simulink model "LDW_mask"  (Simulink 7.6)
settings: Solver=FixedStepDiscrete  StartTime=0.0  StopTime=10  FixedStep=1/100  RelTol=1e-3
undefined symbols (not defined in the file): High, num_targets, slselsubs
libraries: simulink x36, dspobslib x14, viptextngfix x9, dspmtrx3 x7, dspsigops x6, simulink_extras x4, viptransforms x4, dspstat3 x4, dspswit3 x3, dspadpt3 x3, dspindex x2, vipconversions x2
(part 3 of 3)

== system LDW_mask/LDW Model/Subsystem1/Lane Detection/Peak detection/Enable signal generator ==
  Num : Inport
  Assignment : Assignment  NumberOfDimensions=2  IndexOptions=Assign all,Index vector (port)  Indices=-1,1  OutputSizes=1,1
  Constant : Constant  Value=zeros(1, expLaneNum)  VectorParams1D=off  OutDataTypeStr=boolean
  Constant1 : Constant  VectorParams1D=off  OutDataTypeStr=boolean
  For Iterator : ForIterator  ResetStates=reset  IterationSource=external
  Enable : Outport
  wires:
  For Iterator/1 -> Assignment/3
  Constant1/1 -> Assignment/2
  Assignment/1 -> Enable/1
  Constant/1 -> Assignment/1
  Num/1 -> For Iterator/1

== system LDW_mask/LDW Model/Subsystem1/Lane Detection/Peak detection1/Enable signal generator ==
  Num : Inport
  Assignment : Assignment  NumberOfDimensions=2  IndexOptions=Assign all,Index vector (port)  Indices=-1,1  OutputSizes=1,1
  Constant : Constant  Value=zeros(1, expLaneNum)  VectorParams1D=off  OutDataTypeStr=boolean
  Constant1 : Constant  VectorParams1D=off  OutDataTypeStr=boolean
  For Iterator : ForIterator  ResetStates=reset  IterationSource=external
  Enable : Outport
  wires:
  Num/1 -> For Iterator/1
  Constant/1 -> Assignment/1
  Assignment/1 -> Enable/1
  Constant1/1 -> Assignment/2
  For Iterator/1 -> Assignment/3

== system LDW_mask/LDW Model/Subsystem1/Lane Tracking/Matching/Calculate the distances between  the lines found in the current  frame and those in the respository ==
  Count : Inport
  Rep_ref : Inport  Port=2
  Line : Inport  Port=3
  Enable : Inport  Port=4
  For Iterator : ForIterator  ResetStates=reset  IterationLimit=maxLaneNum
  "Select a line from the repository; if it is valid (Count > 0),  Calculate its distance to the input lines." : Subsystem
  Selector1 : Selector  NumberOfDimensions=2  InputPortWidth=3  IndexOptions=Select all,Index vector (port)  Indices=-1,-1  OutputSizes=1
  Dis : Outport
  wires:
  Enable/1 -> "Select a line from the repository; if it is valid (Count > 0),  Calculate its distance to the input lines."/4(Enable)
  For Iterator/1 -> Selector1/2, "Select a line from the repository; if it is valid (Count > 0),  Calculate its distance to the input lines."/1(Idx)
  "Select a line from the repository; if it is valid (Count > 0),  Calculate its distance to the input lines."/1(Dis) -> Dis/1
  Rep_ref/1 -> "Select a line from the repository; if it is valid (Count > 0),  Calculate its distance to the input lines."/2(Rep_ref)
  Line/1 -> "Select a line from the repository; if it is valid (Count > 0),  Calculate its distance to the input lines."/3(Line)
  Count/1 -> Selector1/1
  Selector1/1 -> "Select a line from the repository; if it is valid (Count > 0),  Calculate its distance to the input lines."/Enable

== system LDW_mask/LDW Model/Subsystem1/Lane Tracking/Matching/Find the best  matches between the current  lines and those in the repository ==
  note: In the 1st iteration, find minimum element (corresponds to
      | best matching targets) in the distance matrix. Then, use the
      | updated distance matrix where the minimum elements and
      | their  corresponding rows and columns have been reset.
  note: Reset the column where the
      | minimum element lies on.
  note: Reset the row where the
      | minimum element lies on.
  Dis : Inport
  Add : Sum
  Assignment : Assignment  NumberOfDimensions=2  IndexOptions=Assign all,Index vector (port)  Indices=-1,-1  OutputSizes=1,1
  Assignment1 : Assignment  NumberOfDimensions=2  IndexOptions=Index vector (port),Assign all  Indices=1,-1  OutputSizes=1,1
  Assignment2 : Assignment  NumberOfDimensions=2  IndexOptions=Assign all,Index vector (port)  Indices=-1,-1  OutputSizes=1,1
  Assignment3 : Assignment  NumberOfDimensions=2  IndexOptions=Assign all,Index vector (port)  Indices=-1,-1  OutputSizes=1,1
  Compare To Constant : simulink/Logic and Bit Operations/Compare To Constant  SystemSampleTime=-1  relop=<=  const=1  LogicOutDataTypeMode=boolean  ZeroCross=off
  Constant : Constant  Value=intmax('int16')  VectorParams1D=off  OutDataTypeStr=Inherit: Inherit via back propagation
  Constant1 : Constant  Value=intmax('int16')*ones(1,maxLaneNum, 'int16')  VectorParams1D=off  OutDataTypeStr=Inherit: Inherit via back propagation
  Constant2 : Constant  Value=zeros(2,maxLaneNum)  VectorParams1D=off  OutDataTypeStr=Inherit: Inherit via back propagation
  Data Type  Conversion3 : DataTypeConversion  OutDataTypeStr=int32  SaturateOnIntegerOverflow=on  RndMeth=Zero
  Delay1 : dspsigops/Delay  dly_unit=Samples  delay=1  ic_detail=off  dif_ic_for_ch=off  dif_ic_for_dly=off  ic=0  reset_popup=None
  For Iterator : ForIterator  IterationLimit=expLaneNum
  Minimum : dspstat3/Minimum  DialogController=dspDDGCreate  DialogControllerArgs=DataTag11  fcn=Value and Index  reset=None  indexBase=One  operateOver=Entire input  Dimension=1  colComp=on  operation=minimum  roiEnable=off  roiType=Rectangles  roiPortion=Entire ROI  roiOutput=Individual statistics for each ROI  roiFlag=off  roundingMode=Floor  overflowMode=off
  Reshape : Reshape  OutputDimensionality=Column vector (2-D)
  Selector : Selector  InputPortWidth=2  IndexOptions=Index vector (dialog)  Indices=[2]  OutputSizes=1
  Selector1 : Selector  InputPortWidth=2  IndexOptions=Index vector (dialog)  Indices=[1]  OutputSizes=1
  Switch1 : Switch  Criteria=u2 ~= 0
  Match_list : Outport
  Match_dis : Outport  Port=2
  wires:
  Constant2/1 -> Assignment/1
  Constant1/1 -> Assignment3/1
  Data Type  Conversion3/1 -> Reshape/1
  Compare To Constant/1 -> Switch1/2
  For Iterator/1 -> Compare To Constant/1, Assignment/3, Assignment3/3
  Switch1/1 -> Minimum/1
  Dis/1 -> Assignment2/1, Assignment1/1, Switch1/1
  Delay1/1 -> Switch1/3
  Assignment/1 -> Match_list/1
  Selector/1 -> Assignment2/3
  Selector1/1 -> Assignment1/3
  Assignment1/1 -> Add/1
  Assignment2/1 -> Add/2
  Add/1 -> Delay1/1
  Assignment3/1 -> Match_dis/1
  Minimum/2 -> Data Type  Conversion3/1, Selector/1, Selector1/1
  Minimum/1 -> Assignment3/2
  Constant/1 -> Assignment1/2, Assignment2/2
  Reshape/1 -> Assignment/2

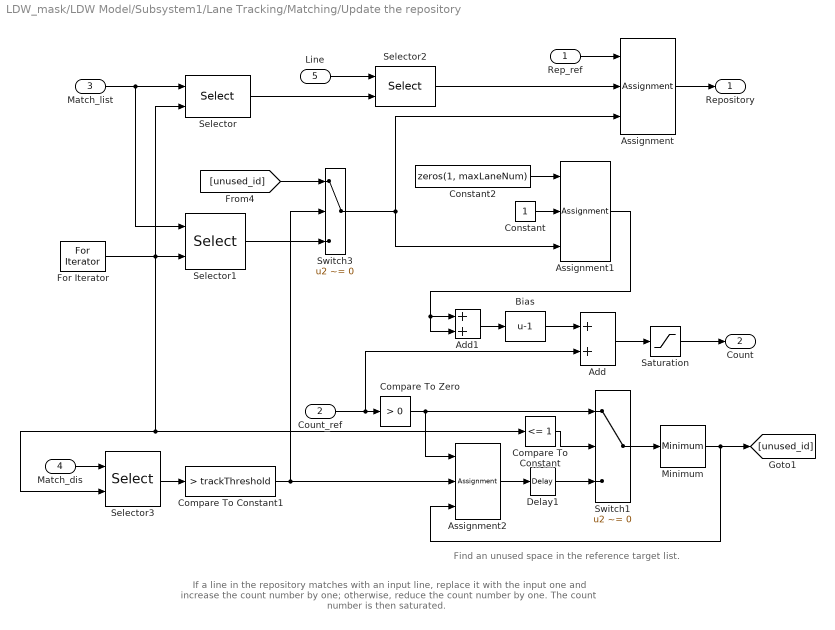
== system LDW_mask/LDW Model/Subsystem1/Lane Tracking/Matching/Update the repository ==
  note: Find an unused space in the reference target list.
  note: If a line in the repository matches with an input line, replace it with the input one and increase the count number by one;
      | otherwise, reduce the count number by one. The count number is then saturated.
  Rep_ref : Inport
  Count_ref : Inport  Port=2
  Match_list : Inport  Port=3
  Match_dis : Inport  Port=4
  Line : Inport  Port=5
  Add : Sum  InputSameDT=on
  Add1 : Sum  OutDataTypeStr=int32  InputSameDT=on
  Assignment : Assignment  NumberOfDimensions=2  IndexOptions=Assign all,Starting index (port)  Indices=-1,-1  OutputSizes=1,1
  Assignment1 : Assignment  NumberOfDimensions=2  IndexOptions=Assign all,Index vector (port)  Indices=-1,-1  OutputSizes=slselsubs([1, num_targets],1),slselsubs([1, num_targets],2)
  Assignment2 : Assignment  IndexOptions=Index vector (port)  Indices=-1  OutputSizes=[1, num_targets]
  Bias : Bias  Bias=-1
  Compare To Constant : simulink/Logic and Bit Operations/Compare To Constant  SystemSampleTime=-1  relop=<=  const=1  LogicOutDataTypeMode=boolean  ZeroCross=off
  Compare To Constant1 : simulink/Logic and Bit Operations/Compare To Constant  SystemSampleTime=-1  relop=>  const=trackThreshold  LogicOutDataTypeMode=boolean  ZeroCross=off
  Compare To Zero : simulink/Logic and Bit Operations/Compare To Zero  SystemSampleTime=-1  relop=>  LogicOutDataTypeMode=boolean  ZeroCross=off
  Constant : Constant  VectorParams1D=off  OutDataTypeStr=Inherit: Inherit via back propagation
  Constant2 : Constant  Value=zeros(1, maxLaneNum)  VectorParams1D=off  OutDataTypeStr=int32
  Delay1 : dspsigops/Delay  dly_unit=Samples  delay=1  ic_detail=off  dif_ic_for_ch=off  dif_ic_for_dly=off  ic=0  reset_popup=None
  For Iterator : ForIterator  ResetStates=reset  IterationLimit=expLaneNum
  Minimum : dspstat3/Minimum  DialogController=dspDDGCreate  DialogControllerArgs=DataTag12  fcn=Index  reset=None  indexBase=One  operateOver=Each row  Dimension=1  colComp=on  operation=minimum  roiEnable=off  roiType=Rectangles  roiPortion=Entire ROI  roiOutput=Individual statistics for each ROI  roiFlag=off  roundingMode=Floor  overflowMode=off
  Saturation : Saturate  UpperLimit=frameFound+frameLost  LowerLimit=0
  Selector : Selector  NumberOfDimensions=2  InputPortWidth=3  IndexOptions=Index vector (dialog),Index vector (port)  Indices=[2],[1]  OutputSizes=1
  Selector1 : Selector  NumberOfDimensions=2  InputPortWidth=3  IndexOptions=Index vector (dialog),Index vector (port)  Indices=[1],[2]  OutputSizes=1
  Selector2 : Selector  NumberOfDimensions=2  InputPortWidth=3  IndexOptions=Select all,Index vector (port)  Indices=-1,1  OutputSizes=1
  Selector3 : Selector  NumberOfDimensions=2  InputPortWidth=3  IndexOptions=Select all,Index vector (port)  Indices=-1,-1  OutputSizes=1
  Switch1 : Switch  Criteria=u2 ~= 0
  Switch3 : Switch  Criteria=u2 ~= 0
  Repository : Outport
  Count : Outport  Port=2
  wires:
  Constant2/1 -> Assignment1/1
  Constant/1 -> Assignment1/2
  Switch3/1 -> Assignment1/3, Assignment/3
  Selector1/1 -> Switch3/3
  Selector/1 -> Selector2/2
  [unused_id] -> Switch3/1
  Compare To Constant1/1 -> Switch3/2, Assignment2/2
  Delay1/1 -> Switch1/3
  Count_ref/1 -> Add/2, Compare To Zero/1
  Switch1/1 -> Minimum/1
  Minimum/1 -> [unused_id], Assignment2/3
  Assignment2/1 -> Delay1/1
  Match_dis/1 -> Selector3/1
  Assignment1/1 -> Add1/1, Add1/2
  Assignment/1 -> Repository/1
  Line/1 -> Selector2/1
  Match_list/1 -> Selector/1, Selector1/1
  Compare To Constant/1 -> Switch1/2
  For Iterator/1 -> Selector3/2, Compare To Constant/1, Selector/2, Selector1/2
  Selector2/1 -> Assignment/2
  Add1/1 -> Bias/1
  Bias/1 -> Add/1
  Add/1 -> Saturation/1
  Compare To Zero/1 -> Switch1/1, Assignment2/1
  Rep_ref/1 -> Assignment/1
  Selector3/1 -> Compare To Constant1/1
  Saturation/1 -> Count/1

== system LDW_mask/LDW Model/Subsystem1/Lane Tracking1/Matching/Calculate the distances between  the lines found in the current  frame and those in the respository ==
  Count : Inport
  Rep_ref : Inport  Port=2
  Line : Inport  Port=3
  Enable : Inport  Port=4
  For Iterator : ForIterator  ResetStates=reset  IterationLimit=maxLaneNum
  "Select a line from the repository; if it is valid (Count > 0),  Calculate its distance to the input lines." : Subsystem
  Selector1 : Selector  NumberOfDimensions=2  InputPortWidth=3  IndexOptions=Select all,Index vector (port)  Indices=-1,-1  OutputSizes=1
  Dis : Outport
  wires:
  Selector1/1 -> "Select a line from the repository; if it is valid (Count > 0),  Calculate its distance to the input lines."/Enable
  Count/1 -> Selector1/1
  Line/1 -> "Select a line from the repository; if it is valid (Count > 0),  Calculate its distance to the input lines."/3(Line)
  Rep_ref/1 -> "Select a line from the repository; if it is valid (Count > 0),  Calculate its distance to the input lines."/2(Rep_ref)
  "Select a line from the repository; if it is valid (Count > 0),  Calculate its distance to the input lines."/1(Dis) -> Dis/1
  For Iterator/1 -> "Select a line from the repository; if it is valid (Count > 0),  Calculate its distance to the input lines."/1(Idx), Selector1/2
  Enable/1 -> "Select a line from the repository; if it is valid (Count > 0),  Calculate its distance to the input lines."/4(Enable)

== system LDW_mask/LDW Model/Subsystem1/Lane Tracking1/Matching/Find the best  matches between the current  lines and those in the repository ==
  note: Reset the row where the
      | minimum element lies on.
  note: Reset the column where the
      | minimum element lies on.
  note: In the 1st iteration, find minimum element (corresponds to
      | best matching targets) in the distance matrix. Then, use the
      | updated distance matrix where the minimum elements and
      | their  corresponding rows and columns have been reset.
  Dis : Inport
  Add : Sum
  Assignment : Assignment  NumberOfDimensions=2  IndexOptions=Assign all,Index vector (port)  Indices=-1,-1  OutputSizes=1,1
  Assignment1 : Assignment  NumberOfDimensions=2  IndexOptions=Index vector (port),Assign all  Indices=1,-1  OutputSizes=1,1
  Assignment2 : Assignment  NumberOfDimensions=2  IndexOptions=Assign all,Index vector (port)  Indices=-1,-1  OutputSizes=1,1
  Assignment3 : Assignment  NumberOfDimensions=2  IndexOptions=Assign all,Index vector (port)  Indices=-1,-1  OutputSizes=1,1
  Compare To Constant : simulink/Logic and Bit Operations/Compare To Constant  SystemSampleTime=-1  relop=<=  const=1  LogicOutDataTypeMode=boolean  ZeroCross=off
  Constant : Constant  Value=intmax('int16')  VectorParams1D=off  OutDataTypeStr=Inherit: Inherit via back propagation
  Constant1 : Constant  Value=intmax('int16')*ones(1,maxLaneNum, 'int16')  VectorParams1D=off  OutDataTypeStr=Inherit: Inherit via back propagation
  Constant2 : Constant  Value=zeros(2,maxLaneNum)  VectorParams1D=off  OutDataTypeStr=Inherit: Inherit via back propagation
  Data Type  Conversion3 : DataTypeConversion  OutDataTypeStr=int32  SaturateOnIntegerOverflow=on  RndMeth=Zero
  Delay1 : dspsigops/Delay  dly_unit=Samples  delay=1  ic_detail=off  dif_ic_for_ch=off  dif_ic_for_dly=off  ic=0  reset_popup=None
  For Iterator : ForIterator  IterationLimit=expLaneNum
  Minimum : dspstat3/Minimum  DialogController=dspDDGCreate  DialogControllerArgs=DataTag14  fcn=Value and Index  reset=None  indexBase=One  operateOver=Entire input  Dimension=1  colComp=on  operation=minimum  roiEnable=off  roiType=Rectangles  roiPortion=Entire ROI  roiOutput=Individual statistics for each ROI  roiFlag=off  roundingMode=Floor  overflowMode=off
  Reshape : Reshape  OutputDimensionality=Column vector (2-D)
  Selector : Selector  InputPortWidth=2  IndexOptions=Index vector (dialog)  Indices=[2]  OutputSizes=1
  Selector1 : Selector  InputPortWidth=2  IndexOptions=Index vector (dialog)  Indices=[1]  OutputSizes=1
  Switch1 : Switch  Criteria=u2 ~= 0
  Match_list : Outport
  Match_dis : Outport  Port=2
  wires:
  Reshape/1 -> Assignment/2
  Constant/1 -> Assignment2/2, Assignment1/2
  Minimum/1 -> Assignment3/2
  Minimum/2 -> Selector1/1, Selector/1, Data Type  Conversion3/1
  Assignment3/1 -> Match_dis/1
  Add/1 -> Delay1/1
  Assignment2/1 -> Add/2
  Assignment1/1 -> Add/1
  Selector1/1 -> Assignment1/3
  Selector/1 -> Assignment2/3
  Assignment/1 -> Match_list/1
  Delay1/1 -> Switch1/3
  Dis/1 -> Switch1/1, Assignment1/1, Assignment2/1
  Switch1/1 -> Minimum/1
  For Iterator/1 -> Assignment3/3, Assignment/3, Compare To Constant/1
  Compare To Constant/1 -> Switch1/2
  Data Type  Conversion3/1 -> Reshape/1
  Constant1/1 -> Assignment3/1
  Constant2/1 -> Assignment/1

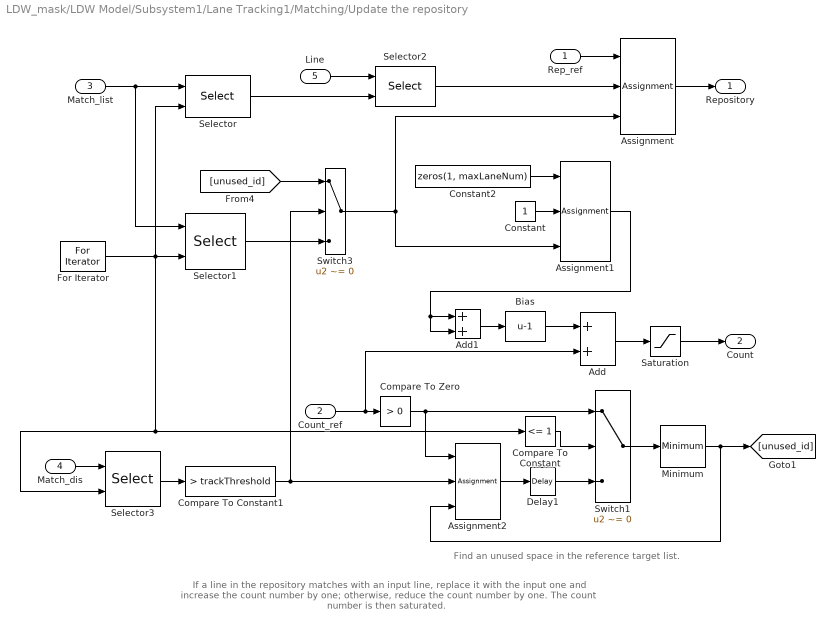
== system LDW_mask/LDW Model/Subsystem1/Lane Tracking1/Matching/Update the repository ==
  note: If a line in the repository matches with an input line, replace it with the input one and increase the count number by one;
      | otherwise, reduce the count number by one. The count number is then saturated.
  note: Find an unused space in the reference target list.
  Rep_ref : Inport
  Count_ref : Inport  Port=2
  Match_list : Inport  Port=3
  Match_dis : Inport  Port=4
  Line : Inport  Port=5
  Add : Sum  InputSameDT=on
  Add1 : Sum  OutDataTypeStr=int32  InputSameDT=on
  Assignment : Assignment  NumberOfDimensions=2  IndexOptions=Assign all,Starting index (port)  Indices=-1,-1  OutputSizes=1,1
  Assignment1 : Assignment  NumberOfDimensions=2  IndexOptions=Assign all,Index vector (port)  Indices=-1,-1  OutputSizes=slselsubs([1, num_targets],1),slselsubs([1, num_targets],2)
  Assignment2 : Assignment  IndexOptions=Index vector (port)  Indices=-1  OutputSizes=[1, num_targets]
  Bias : Bias  Bias=-1
  Compare To Constant : simulink/Logic and Bit Operations/Compare To Constant  SystemSampleTime=-1  relop=<=  const=1  LogicOutDataTypeMode=boolean  ZeroCross=off
  Compare To Constant1 : simulink/Logic and Bit Operations/Compare To Constant  SystemSampleTime=-1  relop=>  const=trackThreshold  LogicOutDataTypeMode=boolean  ZeroCross=off
  Compare To Zero : simulink/Logic and Bit Operations/Compare To Zero  SystemSampleTime=-1  relop=>  LogicOutDataTypeMode=boolean  ZeroCross=off
  Constant : Constant  VectorParams1D=off  OutDataTypeStr=Inherit: Inherit via back propagation
  Constant2 : Constant  Value=zeros(1, maxLaneNum)  VectorParams1D=off  OutDataTypeStr=int32
  Delay1 : dspsigops/Delay  dly_unit=Samples  delay=1  ic_detail=off  dif_ic_for_ch=off  dif_ic_for_dly=off  ic=0  reset_popup=None
  For Iterator : ForIterator  ResetStates=reset  IterationLimit=expLaneNum
  Minimum : dspstat3/Minimum  DialogController=dspDDGCreate  DialogControllerArgs=DataTag15  fcn=Index  reset=None  indexBase=One  operateOver=Each row  Dimension=1  colComp=on  operation=minimum  roiEnable=off  roiType=Rectangles  roiPortion=Entire ROI  roiOutput=Individual statistics for each ROI  roiFlag=off  roundingMode=Floor  overflowMode=off
  Saturation : Saturate  UpperLimit=frameFound+frameLost  LowerLimit=0
  Selector : Selector  NumberOfDimensions=2  InputPortWidth=3  IndexOptions=Index vector (dialog),Index vector (port)  Indices=[2],[1]  OutputSizes=1
  Selector1 : Selector  NumberOfDimensions=2  InputPortWidth=3  IndexOptions=Index vector (dialog),Index vector (port)  Indices=[1],[2]  OutputSizes=1
  Selector2 : Selector  NumberOfDimensions=2  InputPortWidth=3  IndexOptions=Select all,Index vector (port)  Indices=-1,1  OutputSizes=1
  Selector3 : Selector  NumberOfDimensions=2  InputPortWidth=3  IndexOptions=Select all,Index vector (port)  Indices=-1,-1  OutputSizes=1
  Switch1 : Switch  Criteria=u2 ~= 0
  Switch3 : Switch  Criteria=u2 ~= 0
  Repository : Outport
  Count : Outport  Port=2
  wires:
  Saturation/1 -> Count/1
  Selector3/1 -> Compare To Constant1/1
  Rep_ref/1 -> Assignment/1
  Compare To Zero/1 -> Assignment2/1, Switch1/1
  Add/1 -> Saturation/1
  Bias/1 -> Add/1
  Add1/1 -> Bias/1
  Selector2/1 -> Assignment/2
  For Iterator/1 -> Selector1/2, Selector/2, Compare To Constant/1, Selector3/2
  Compare To Constant/1 -> Switch1/2
  Match_list/1 -> Selector1/1, Selector/1
  Line/1 -> Selector2/1
  Assignment/1 -> Repository/1
  Assignment1/1 -> Add1/2, Add1/1
  Match_dis/1 -> Selector3/1
  Assignment2/1 -> Delay1/1
  Minimum/1 -> Assignment2/3, [unused_id]
  Switch1/1 -> Minimum/1
  Count_ref/1 -> Compare To Zero/1, Add/2
  Delay1/1 -> Switch1/3
  Compare To Constant1/1 -> Assignment2/2, Switch3/2
  [unused_id] -> Switch3/1
  Selector/1 -> Selector2/2
  Selector1/1 -> Switch3/3
  Switch3/1 -> Assignment/3, Assignment1/3
  Constant/1 -> Assignment1/2
  Constant2/1 -> Assignment1/1

== system LDW_mask/LDW Model/Subsystem1/Output/Subsystem/Draw  Polygon ==
  inPts : Inport
  RGB : Inport  Port=2
  Enable : EnablePort  PropagateVarSize=During execution
  DrawShapes : viptextngfix/Draw Shapes  DialogController=vipDDGCreate  DialogControllerArgs=DataTag21  shape=Polygons  fill=on  fillClrSource=Specify via dialog  display=User-specified value  intensity=200  color=[0 1 1]  opacity=0.2  viewport=Entire image  antialiasing=off  inType=Obsolete  imagePorts=One multidimensional signal  prodOutputMode=Binary point scaling  prodOutputWordLength=32  prodOutputFracLength=14  memoryMode=Specify word length  memoryWordLength=16  memoryFracLength=14  roundingMode=Floor  overflowMode=off
  Line to Polygon Coordinates : Subsystem
  RGBout : Outport
  wires:
  RGB/1 -> DrawShapes/1
  DrawShapes/1 -> RGBout/1
  inPts/1 -> Line to Polygon Coordinates/1(Pts_line)
  Line to Polygon Coordinates/1(Pts_polygon) -> DrawShapes/2

== system LDW_mask/LDW Model/Subsystem1/Output/Subsystem/Draw Color and Marker Type ==
  Image : Inport
  Ldis : Inport  Port=2
  Rdis : Inport  Port=3
  Bias : Bias  Bias=-1
  Bias3 : Bias  Bias=-1
  Constant : Constant  Value=[1 0 0]  OutDataTypeStr=single  SampleTime=vfq
  Constant1 : Constant  Value=[1 0 0]  OutDataTypeStr=single  SampleTime=vfq
  Constant6 : Constant  Value=[1 1 0]  OutDataTypeStr=single  SampleTime=vfq
  Constant7 : Constant  Value=[1 1 0]  OutDataTypeStr=single  SampleTime=vfq
  Gain : Gain  Gain=3.5/480  OutDataTypeStr=double
  Gain1 : Gain  Gain=3.5/480  OutDataTypeStr=double
  Insert Text: Left Distance : viptextngfix/Insert Text  DialogController=vipDDGCreate  DialogControllerArgs=DataTag22  inputType=Obsolete  theText=['Distance: %4.1f m']  fontFace=LucidaTypewriterBold  dummyVar1=0  blockFontSize=14  antiAliased=on  getTextLocFrom=Specify via dialog  textLoc=[355 10]  getTextColorFrom=Input port  textColor=[1 1 1]  getTextIntensityFrom=Specify via dialog  textIntensity=0  getTextOpacityFrom=Specify via dialog  textOpacity=1  dummyVar2=0  dummyVar3=0  dummyVar4=0  imagePorts=One multidimensional signal  isInputTransposed=off
  Insert Text: Right Distance : viptextngfix/Insert Text  DialogController=vipDDGCreate  DialogControllerArgs=DataTag23  inputType=Obsolete  theText=['Distance: %4.1f m']  fontFace=LucidaTypewriterBold  dummyVar1=0  blockFontSize=14  antiAliased=on  getTextLocFrom=Specify via dialog  textLoc=[355 370]  getTextColorFrom=Input port  textColor=[1 1 1]  getTextIntensityFrom=Specify via dialog  textIntensity=0  getTextOpacityFrom=Specify via dialog  textOpacity=1  dummyVar2=0  dummyVar3=0  dummyVar4=0  imagePorts=One multidimensional signal  isInputTransposed=off
  Switch2 : Switch
  Switch3 : Switch
  Out : Outport
  wires:
  Insert Text: Left Distance/1 -> Insert Text: Right Distance/1
  Insert Text: Right Distance/1 -> Out/1
  Gain/1 -> Bias/1
  Gain1/1 -> Bias3/1
  Ldis/1 -> Gain/1
  Rdis/1 -> Gain1/1
  Constant1/1 -> Switch3/3
  Bias/1 -> Switch3/2, Insert Text: Left Distance/2
  Bias3/1 -> Switch2/2, Insert Text: Right Distance/2
  Constant/1 -> Switch2/3
  Switch2/1 -> Insert Text: Right Distance/3
  Constant6/1 -> Switch3/1
  Image/1 -> Insert Text: Left Distance/1
  Constant7/1 -> Switch2/1
  Switch3/1 -> Insert Text: Left Distance/3

== system LDW_mask/LDW Model/Subsystem1/Lane Tracking/Matching/Calculate the distances between  the lines found in the current  frame and those in the respository/Select a line from the repository; if it is valid (Count > 0),  Calculate its distance to the input lines. ==
  Idx : Inport
  Rep_ref : Inport  Port=2
  Line : Inport  Port=3
  Enable : Inport  Port=4
  EnablePort : EnablePort  StatesWhenEnabling=reset  PropagateVarSize=During execution
  Assignment : Assignment  NumberOfDimensions=2  IndexOptions=Index vector (port),Assign all  Indices=-1,-1  OutputSizes=1,1
  Calculate the distances between  the chosen line in the repository  and all input lines. : Subsystem  TreatAsAtomicUnit=on
  Constant2 : Constant  Value=intmax('int16') * ones(maxLaneNum,'int16')  VectorParams1D=off  OutDataTypeStr=int32
  Selector1 : Selector  NumberOfDimensions=2  InputPortWidth=3  IndexOptions=Index vector (port),Select all  Indices=-1,-1  OutputSizes=1
  Selector2 : Selector  NumberOfDimensions=2  InputPortWidth=3  IndexOptions=Select all,Index vector (port)  Indices=-1,-1  OutputSizes=1
  Dis : Outport
  wires:
  Rep_ref/1 -> Selector2/1
  Enable/1 -> Calculate the distances between  the chosen line in the repository  and all input lines./4(Enable)
  Selector2/1 -> Calculate the distances between  the chosen line in the repository  and all input lines./2(Rep_ref)
  Line/1 -> Calculate the distances between  the chosen line in the repository  and all input lines./3(Line)
  Selector1/1 -> Calculate the distances between  the chosen line in the repository  and all input lines./1(Dis)
  Idx/1 -> Selector2/2, Assignment/3, Selector1/2
  Assignment/1 -> Dis/1
  Calculate the distances between  the chosen line in the repository  and all input lines./1(Dis_out) -> Assignment/2
  Constant2/1 -> Selector1/1, Assignment/1

== system LDW_mask/LDW Model/Subsystem1/Lane Tracking1/Matching/Calculate the distances between  the lines found in the current  frame and those in the respository/Select a line from the repository; if it is valid (Count > 0),  Calculate its distance to the input lines. ==
  Idx : Inport
  Rep_ref : Inport  Port=2
  Line : Inport  Port=3
  Enable : Inport  Port=4
  EnablePort : EnablePort  StatesWhenEnabling=reset  PropagateVarSize=During execution
  Assignment : Assignment  NumberOfDimensions=2  IndexOptions=Index vector (port),Assign all  Indices=-1,-1  OutputSizes=1,1
  Calculate the distances between  the chosen line in the repository  and all input lines. : Subsystem  TreatAsAtomicUnit=on
  Constant2 : Constant  Value=intmax('int16') * ones(maxLaneNum,'int16')  VectorParams1D=off  OutDataTypeStr=int32
  Selector1 : Selector  NumberOfDimensions=2  InputPortWidth=3  IndexOptions=Index vector (port),Select all  Indices=-1,-1  OutputSizes=1
  Selector2 : Selector  NumberOfDimensions=2  InputPortWidth=3  IndexOptions=Select all,Index vector (port)  Indices=-1,-1  OutputSizes=1
  Dis : Outport
  wires:
  Constant2/1 -> Assignment/1, Selector1/1
  Calculate the distances between  the chosen line in the repository  and all input lines./1(Dis_out) -> Assignment/2
  Assignment/1 -> Dis/1
  Idx/1 -> Selector1/2, Assignment/3, Selector2/2
  Selector1/1 -> Calculate the distances between  the chosen line in the repository  and all input lines./1(Dis)
  Line/1 -> Calculate the distances between  the chosen line in the repository  and all input lines./3(Line)
  Selector2/1 -> Calculate the distances between  the chosen line in the repository  and all input lines./2(Rep_ref)
  Enable/1 -> Calculate the distances between  the chosen line in the repository  and all input lines./4(Enable)
  Rep_ref/1 -> Selector2/1

== system LDW_mask/LDW Model/Subsystem1/Output/Subsystem/Draw  Polygon/Line to Polygon Coordinates ==
  note: r1   R1
      | c1   C1
      | r2   R2
      | c2   C2
  note: r1
      | c1
  note: R1
      | C1
  note: (r1,c1)
      |                        /
      |                    /
      |               /
      |          /
      | (r2,c2)
  note: (R1,C1)
      |  \
      |        \
      |            \
      |                  \
      |                        (R2,C2)
  note: R2
      | C2
  note: r1
      | c1
      | ----
      | r2
      | c2
      | ----
      | r2     or   239
      | c2     or    0
      | ------
      | R2    or    239
      | C2    or    359
      | -----
      | R2
      | C2
      | -----
      | R1
      | C1
  note: r2
      | c2
  note: r2
      | c2
  note: r2     or   239
      | c2     or    0
  note: R2
      | C2
  note: R2    or    239
      | C2    or    359
  Pts_line : Inport
  DSP Constant : dspobslib/DSP Constant  SystemSampleTime=-1  Value=[239 0]'  SampleMode=Discrete  discreteOutput=Sample-based  continuousOutput=Sample-based  sampTime=vfq  framePeriod=2  dataType=int32  isSigned=on  wordLen=16  udDataType=sfix(16)  fracBitsMode=Best precision  numFracBits=15  InterpretAs1D=-inf  Ts=-inf  FramebasedOutput=-inf
  DSP Constant2 : dspobslib/DSP Constant  SystemSampleTime=-1  Value=[239 359]'  SampleMode=Discrete  discreteOutput=Sample-based  continuousOutput=Sample-based  sampTime=vfq  framePeriod=2  dataType=int32  isSigned=on  wordLen=16  udDataType=sfix(16)  fracBitsMode=Best precision  numFracBits=15  InterpretAs1D=-inf  Ts=-inf  FramebasedOutput=-inf
  Matrix Concatenation6 : Concatenate  NumInputs=6  Mode=Multidimensional array
  Selector : Selector  NumberOfDimensions=2  InputPortWidth=3  IndexOptions=Index vector (dialog),Index vector (dialog)  Indices=3:4,2  OutputSizes=1
  Selector1 : Selector  NumberOfDimensions=2  InputPortWidth=3  IndexOptions=Index vector (dialog),Index vector (dialog)  Indices=1:2,1  OutputSizes=1
  Selector2 : Selector  NumberOfDimensions=2  InputPortWidth=3  IndexOptions=Index vector (dialog),Index vector (dialog)  Indices=1:2,2  OutputSizes=1
  Selector3 : Selector  InputPortWidth=2  IndexOptions=Index vector (dialog)  Indices=1  OutputSizes=1
  Selector4 : Selector  NumberOfDimensions=2  InputPortWidth=3  IndexOptions=Index vector (dialog),Index vector (dialog)  Indices=3:4,1  OutputSizes=1
  Selector5 : Selector  InputPortWidth=2  IndexOptions=Index vector (dialog)  Indices=1  OutputSizes=1
  Switch : Switch  Threshold=239
  Switch1 : Switch  Threshold=239
  Pts_polygon : Outport
  wires:
  Selector1/1 -> Matrix Concatenation6/1
  Selector/1 -> Switch1/1, Selector5/1, Matrix Concatenation6/5
  Matrix Concatenation6/1 -> Pts_polygon/1
  Selector3/1 -> Switch/2  "r2"
  Selector4/1 -> Switch/1, Selector3/1, Matrix Concatenation6/2
  DSP Constant/1 -> Switch/3
  Selector5/1 -> Switch1/2  "R2"
  DSP Constant2/1 -> Switch1/3
  Selector2/1 -> Matrix Concatenation6/6
  Switch/1 -> Matrix Concatenation6/3
  Switch1/1 -> Matrix Concatenation6/4
  Pts_line/1 -> Selector1/1, Selector4/1, Selector/1, Selector2/1

== system LDW_mask/LDW Model/Subsystem1/Lane Tracking/Matching/Calculate the distances between  the lines found in the current  frame and those in the respository/Select a line from the repository; if it is valid (Count > 0),  Calculate its distance to the input lines./Calculate the distances between  the chosen line in the repository  and all input lines. ==
  note: Calculate the distance between the chosen line in the repository and every input line.
  Dis : Inport
  Rep_ref : Inport  Port=2
  Line : Inport  Port=3
  Enable : Inport  Port=4
  Assignment : Assignment  IndexOptions=Index vector (port)  Indices=1  OutputSizes=[1 1]
  Constant : Constant  Value=intmax('int16')  VectorParams1D=off  OutDataTypeStr=int32
  Difference between  two lines : Subsystem
  For Iterator : ForIterator  ResetStates=reset  IterationLimit=expLaneNum
  Selector1 : Selector  NumberOfDimensions=2  InputPortWidth=3  IndexOptions=Select all,Index vector (port)  Indices=-1,-1  OutputSizes=1
  Selector2 : Selector  NumberOfDimensions=2  InputPortWidth=3  IndexOptions=Select all,Index vector (port)  Indices=-1,-1  OutputSizes=1
  Switch1 : Switch  Criteria=u2 ~= 0
  Dis_out : Outport
  wires:
  Selector1/1 -> Difference between  two lines/2(Line_2)
  Constant/1 -> Switch1/3
  Difference between  two lines/1(Dis) -> Switch1/1
  Selector2/1 -> Switch1/2, Difference between  two lines/Enable
  Enable/1 -> Selector2/1
  Line/1 -> Selector1/1
  For Iterator/1 -> Selector1/2, Selector2/2, Assignment/3
  Rep_ref/1 -> Difference between  two lines/1(Line_1)
  Dis/1 -> Assignment/1
  Assignment/1 -> Dis_out/1
  Switch1/1 -> Assignment/2

== system LDW_mask/LDW Model/Subsystem1/Lane Tracking1/Matching/Calculate the distances between  the lines found in the current  frame and those in the respository/Select a line from the repository; if it is valid (Count > 0),  Calculate its distance to the input lines./Calculate the distances between  the chosen line in the repository  and all input lines. ==
  note: Calculate the distance between the chosen line in the repository and every input line.
  Dis : Inport
  Rep_ref : Inport  Port=2
  Line : Inport  Port=3
  Enable : Inport  Port=4
  Assignment : Assignment  IndexOptions=Index vector (port)  Indices=1  OutputSizes=[1 1]
  Constant : Constant  Value=intmax('int16')  VectorParams1D=off  OutDataTypeStr=int32
  Difference between  two lines : Subsystem
  For Iterator : ForIterator  ResetStates=reset  IterationLimit=expLaneNum
  Selector1 : Selector  NumberOfDimensions=2  InputPortWidth=3  IndexOptions=Select all,Index vector (port)  Indices=-1,-1  OutputSizes=1
  Selector2 : Selector  NumberOfDimensions=2  InputPortWidth=3  IndexOptions=Select all,Index vector (port)  Indices=-1,-1  OutputSizes=1
  Switch1 : Switch  Criteria=u2 ~= 0
  Dis_out : Outport
  wires:
  Switch1/1 -> Assignment/2
  Assignment/1 -> Dis_out/1
  Dis/1 -> Assignment/1
  Rep_ref/1 -> Difference between  two lines/1(Line_1)
  For Iterator/1 -> Assignment/3, Selector2/2, Selector1/2
  Enable/1 -> Selector2/1
  Selector2/1 -> Difference between  two lines/Enable, Switch1/2
  Difference between  two lines/1(Dis) -> Switch1/1
  Constant/1 -> Switch1/3
  Selector1/1 -> Difference between  two lines/2(Line_2)
  Line/1 -> Selector1/1

== system LDW_mask/LDW Model/Subsystem1/Lane Tracking/Matching/Calculate the distances between  the lines found in the current  frame and those in the respository/Select a line from the repository; if it is valid (Count > 0),  Calculate its distance to the input lines./Calculate the distances between  the chosen line in the repository  and all input lines./Difference between  two lines ==
  note: Distance between two lines equals to
      | abs( Rho1 - Rho2) + abs( Theta1 - Theta2) * estImageSize,
      | where estImageSize is the estimated size of the image.
  Line_1 : Inport
  Line_2 : Inport  Port=2
  Enable : EnablePort  PropagateVarSize=During execution
  Abs : Abs
  Abs1 : Abs
  Add1 : Sum  Inputs=+-  OutDataTypeStr=int32
  Add7 : Sum  OutDataTypeStr=Inherit: Same as first input
  Add8 : Sum  Inputs=+-
  Constant : Constant
  Constant1 : Constant  Value=2
  Gain : Gain  Gain=distanceMetricWeight  OutDataTypeStr=Inherit: Inherit via back propagation
  Rho_1 : Selector  InputPortWidth=2  IndexOptions=Index vector (dialog)  Indices=1  OutputSizes=1
  Rho_2 : Selector  InputPortWidth=2  IndexOptions=Index vector (port)  Indices=1  OutputSizes=1
  Theta_1 : Selector  InputPortWidth=2  IndexOptions=Index vector (dialog)  Indices=2  OutputSizes=1
  Theta_2 : Selector  InputPortWidth=2  IndexOptions=Index vector (port)  Indices=2  OutputSizes=1
  Dis : Outport
  wires:
  Line_1/1 -> Rho_1/1, Theta_1/1
  Line_2/1 -> Rho_2/1, Theta_2/1
  Theta_1/1 -> Add8/1
  Theta_2/1 -> Add8/2
  Add8/1 -> Abs/1
  Add7/1 -> Dis/1
  Abs/1 -> Gain/1
  Add1/1 -> Abs1/1
  Rho_1/1 -> Add1/1
  Rho_2/1 -> Add1/2
  Abs1/1 -> Add7/1
  Gain/1 -> Add7/2
  Constant/1 -> Rho_2/2
  Constant1/1 -> Theta_2/2

== system LDW_mask/LDW Model/Subsystem1/Lane Tracking1/Matching/Calculate the distances between  the lines found in the current  frame and those in the respository/Select a line from the repository; if it is valid (Count > 0),  Calculate its distance to the input lines./Calculate the distances between  the chosen line in the repository  and all input lines./Difference between  two lines ==
  note: Distance between two lines equals to
      | abs( Rho1 - Rho2) + abs( Theta1 - Theta2) * estImageSize,
      | where estImageSize is the estimated size of the image.
  Line_1 : Inport
  Line_2 : Inport  Port=2
  Enable : EnablePort  PropagateVarSize=During execution
  Abs : Abs
  Abs1 : Abs
  Add1 : Sum  Inputs=+-  OutDataTypeStr=int32
  Add7 : Sum  OutDataTypeStr=Inherit: Same as first input
  Add8 : Sum  Inputs=+-
  Constant : Constant
  Constant1 : Constant  Value=2
  Gain : Gain  Gain=distanceMetricWeight  OutDataTypeStr=Inherit: Inherit via back propagation
  Rho_1 : Selector  InputPortWidth=2  IndexOptions=Index vector (dialog)  Indices=1  OutputSizes=1
  Rho_2 : Selector  InputPortWidth=2  IndexOptions=Index vector (port)  Indices=1  OutputSizes=1
  Theta_1 : Selector  InputPortWidth=2  IndexOptions=Index vector (dialog)  Indices=2  OutputSizes=1
  Theta_2 : Selector  InputPortWidth=2  IndexOptions=Index vector (port)  Indices=2  OutputSizes=1
  Dis : Outport
  wires:
  Constant1/1 -> Theta_2/2
  Constant/1 -> Rho_2/2
  Gain/1 -> Add7/2
  Abs1/1 -> Add7/1
  Rho_2/1 -> Add1/2
  Rho_1/1 -> Add1/1
  Add1/1 -> Abs1/1
  Abs/1 -> Gain/1
  Add7/1 -> Dis/1
  Add8/1 -> Abs/1
  Theta_2/1 -> Add8/2
  Theta_1/1 -> Add8/1
  Line_2/1 -> Theta_2/1, Rho_2/1
  Line_1/1 -> Theta_1/1, Rho_1/1

== matlab function LDW Model/Subsystem1/Departure Warning/Depature detection/subsystem/Combine Left Right Departure ==
  data: curMsg input double; prevMsg input int8; outMsg output double; numNormalDrivenFrames input double
function outMsg=CombineLeftRightDeparture(curMsg, prevMsg, numNormalDrivenFrames)  

% It combines left-right departure to left departure
%         and right-left departure to right departure
% It utilizes the fact that there must be at least 4 frames of normal driving 
% between a left departure warning and a right departure warning

%RIGHT_DEP=0; NORMAL=1; LEFT_DEP=2
NORMAL = int8(1);

if curMsg == NORMAL
    outMsg = NORMAL;
else % curMsg == RIGHT_DEP  || curMsg == LEFT_DEP
    if (numNormalDrivenFrames < int32(6))
        % use the previous message
        outMsg = prevMsg;        
    else
        outMsg = curMsg;
    end        
end

== matlab function LDW Model/Subsystem1/Departure Warning/Subsystem3/Embedded MATLAB Function ==
  data: pts_in input double; dist_in input double; pts_out output double; dist_out output double; pts_prev input int32; dist_prev input double; limit_down parameter double; limit_up parameter double
function [pts_out, dist_out] = fcn(pts_in, dist_in, pts_prev, dist_prev, limit_down, limit_up)
%#eml

pts_out = pts_in;
dist_out = dist_in;

pts_mid = double(pts_in);
alpha_rad = atan2(pts_mid(3)-pts_mid(1),pts_mid(4)-pts_mid(2));
alpha = alpha_rad * 180/pi;

% limit_down = 140;
% limit_up = 160;

if (alpha < limit_down) || (alpha >= limit_up)
    pts_out = pts_prev;
    dist_out = dist_prev;
end

end

== matlab function LDW Model/Subsystem1/Departure Warning/Subsystem3/Embedded MATLAB Function1 ==
  data: pts_in input double; dist_in input double; pts_out output double; dist_out output double; pts_prev input double; dist_prev input double; limit_down parameter double; limit_up parameter double
function [pts_out, dist_out] = fcn(pts_in, dist_in, pts_prev, dist_prev, limit_down, limit_up)
%#eml

pts_out = pts_in;
dist_out = dist_in;

pts_mid = double(pts_in);
alpha_rad = atan2(pts_mid(3)-pts_mid(1),pts_mid(4)-pts_mid(2));
alpha = alpha_rad * 180/pi;

% limit_down = 140;
% limit_up = 160;

if (alpha < limit_down) || (alpha >= limit_up)
    pts_out = pts_prev;
    dist_out = dist_prev;
end

end

== matlab function LDW Model/Subsystem1/Departure Warning/Depature detection1/subsystem/Combine Left Right Departure ==
  data: curMsg input double; prevMsg input int8; outMsg output double; numNormalDrivenFrames input double
function outMsg=CombineLeftRightDeparture(curMsg, prevMsg, numNormalDrivenFrames)  

% It combines left-right departure to left departure
%         and right-left departure to right departure
% It utilizes the fact that there must be at least 4 frames of normal driving 
% between a left departure warning and a right departure warning

%RIGHT_DEP=0; NORMAL=1; LEFT_DEP=2
NORMAL = int8(1);

if curMsg == NORMAL
    outMsg = NORMAL;
else % curMsg == RIGHT_DEP  || curMsg == LEFT_DEP
    if (numNormalDrivenFrames < int32(4))
        % use the previous message
        outMsg = prevMsg;        
    else
        outMsg = curMsg;
    end        
end

== matlab function LDW Model/Subsystem1/Departure Warning/Subsystem/MATLAB Function3 ==
  data: L_pts input double; swch output double; R_pts input double; limit_down parameter double; limit_up parameter double
function swch   = fcn(L_pts, R_pts, limit_down, limit_up)
%#eml

L=double(L_pts);
R=double(R_pts);

delta = R(2)-L(2);

%if R(2)-L(2) >= 200 && R(2)-L(2) <= 250
%if R(2)-L(2) >= 160 && R(2)-L(2) <= 190
%if R(2)-L(2) >= 130 && R(2)-L(2) <= 180
if (delta >= limit_down) && (delta <= limit_up)
    swch=1;
else
    swch=2;
end

if R(2) >= 498
    swch=1;
end

if L(2) < 2
    swch=1;
end

end

== matlab function LDW Model/Subsystem1/Lane Detection/Embedded MATLAB Function ==
  data: u input double; y output double size=[2, 2]
function y = fcn(u)
%#eml
y = u;
if isempty(y)
    y = single([0 0; 0 0]);
end

== matlab function LDW Model/Subsystem1/Departure Warning/Subsystem2/MATLAB Function ==
  data: pts input double; Beta output double
function Beta  = fcn(pts)
%#codegen

B=double(pts);
% Alpha = atan2(B(3)-B(1),B(4)-B(2));
Beta = atan2(80-B(1),250-B(2));

end

== matlab function LDW Model/Subsystem1/Input/MATLAB Function ==
  data: u input double; y output double
function y = fcn(u)
%#codegen

y = fliplr(u);
end

== matlab function LDW Model/Subsystem1/Departure Warning/Subsystem2/MATLAB Function1 ==
  data: pts input double; Beta output double
function Beta  = fcn(pts)
%#codegen

B=double(pts);
% Alpha = atan2(B(3)-B(1),B(4)-B(2));
Beta = atan2(80-B(1),250-B(2));

end

== matlab function LDW Model/Subsystem1/Departure Warning/Subsystem2/MATLAB Function2 ==
  data: L_pts input double; dis1 output double; R_pts input double; dis2 output double
function [dis1, dis2] = fcn(L_pts, R_pts)
%#codegen

L=double(L_pts);
R=double(R_pts);
dis1 = sqrt(real([L(1)-R(3); L(2)-R(4)].'*[L(1)-R(3); L(2)-R(4)]));
dis2 = sqrt(real([R(1)-L(3); R(2)-L(4)].'*[R(1)-L(3); R(2)-L(4)]));

end

== matlab function LDW Model/Subsystem1/Departure Warning/Subsystem2/MATLAB Function3 ==
  data: L_pts input double; R_pts input double; angle output double; imgSize parameter double; numRows parameter double
function angle  = fcn(L_pts, R_pts, imgSize, numRows)
%#codegen
H=(imgSize(1)-15)-numRows+1;
L=double(L_pts);
R=double(R_pts);
mpts=(R(4)+ L(4))/2;
X=imgSize(2)/2;
angle = -atan2(mpts-X, H); 
%{
if R(2)-L(2) >= 200 && R(2)-L(2) <= 250
    swch=int32(1);
else
    swch=int32(2);
end
if R(2) >= 498
    swch=int32(1);
end
if L(2) < 2
    swch=int32(1);
end
%}

== matlab function LDW Model/Subsystem1/Lane Detection/Embedded MATLAB Function1 ==
  data: u input double; y output double size=[2, 2]
function y = fcn(u)
%#eml
y = u;
if isempty(y)
    y = single([0 0; 0 0]);
end

== matlab function LDW Model/Subsystem1/Lane Detection/MATLAB Function ==
  data: u input double; y output double
function y = fcn(u)
%#codegen

y = fliplr(u);
end
